simulink model "AFEsimpleModifsPV2"  (R2013a)
settings: Solver=FixedStepDiscrete  SolverMode=SingleTasking  StartTime=0.0  StopTime=5  FixedStep=Tpas  RelTol=1e-3
InitFcn:
  |  AFEsimpleparaDT1
values from neighbouring files (symbols this model uses):
  Freq = 50    [AFE_2L_RC_param_DT1.m]    (also in AFE_FV_Params.m; AFE_PontHPV2.m; AFEsimplepara.m; AFEsimpleparaDT1.m)
  hys = 100    [AFE_2L_RC_param_DT1.m]    (also in AFE_FV_Params.m = 150; AFE_PontHPV2.m = 150; AFEsimplepara.m = 0.1; AFEsimpleparaDT1.m)
  I = (P+Numd(2)/Dend(1))/Ts    [AFE_2L_RC_param_DT1.m]    (also in AFE_PontHPV2.m; AFEsimpleparaDT1.m; AFEsimpleparaPV2.m; initAFE_PontHPV3.m)
  Imax = 1300    [AFE_2L_RC_param_DT1.m]    (also in AFE_FV_Params.m = 1500; AFEsimpleparaDT1.m = 5000; AFEsimpleparaPV2.m = 5000)
  Lac = 8.1487e-04    (= 0.00081487)    [AFE_2L_RC_param_DT1.m]    (also in AFE_FV_Params.m; AFE_PontHPV2.m; AFEsimplepara.m = 0.002; AFEsimpleparaDT1.m)
  P = Numd(1)/Dend(1)    [AFE_2L_RC_param_DT1.m]    (also in AFE_PontHPV2.m; AFEsimpleparaDT1.m; AFEsimpleparaPV2.m; initAFE_PontHPV3.m)
  Rac = 2.5    [AFEsimplepara.m]
  Tpas = 5e-5    (= 5e-05)    [AFE_2L_RC_param_DT1.m]    (also in AFE_FV_Params.m; AFE_PontHPV2.m = 3e-06; AFEsimplepara.m = 1e-05; AFEsimpleparaDT1.m)
  Vac = 2000    [AFE_2L_RC_param_DT1.m]    (also in AFE_FV_Params.m; AFE_PontHPV2.m; AFEsimplepara.m; AFEsimpleparaDT1.m)
libraries: powerlib x16, powerlib_meascontrol x8, simulink x5
settings Model: Creator=LiberT  LastModifiedBy=Daniel
settings DataIOCC: SignalLoggingSaveFormat=ModelDataLogs
settings OptimizationCC: ExpressionDepthLimit=2147483647
settings DebuggingCC: MultiTaskDSMMsg=warning  MultiTaskCondExecSysMsg=none  FcnCallInpInsideContextMsg=EnableAllAsWarning  StrictBusMsg=None
settings RTWCC: IncludeERTFirstTime=on

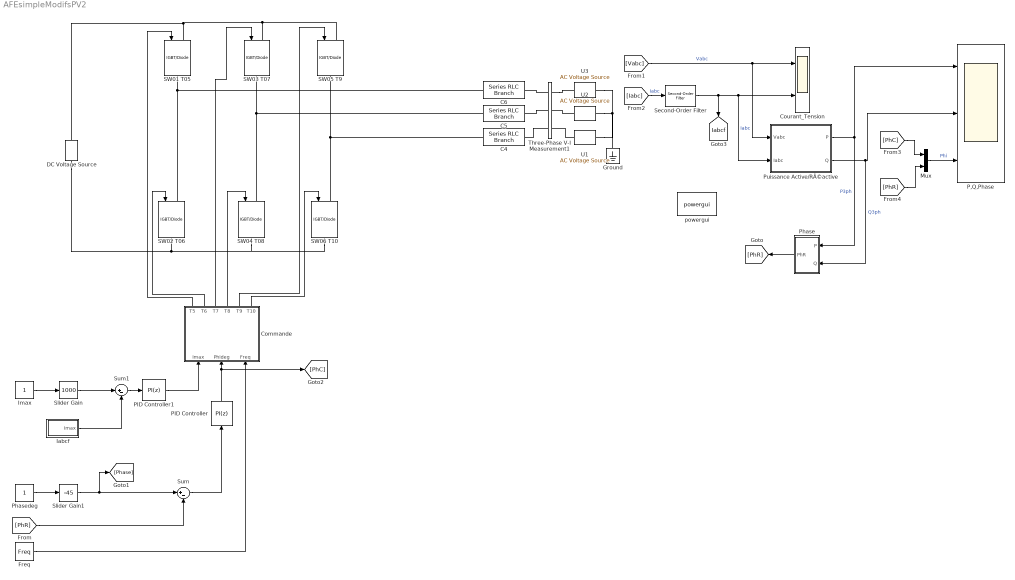
== system AFEsimpleModifsPV2 ==
  C4 : powerlib/Elements/Series RLC Branch  LConnTagsString=__new0  RConnTagsString=__new0  BranchType=L  Resistance=Rac  Inductance=Lac  SetiL0=off  InitialCurrent=0  Capacitance=300e-3  Setx0=off  InitialVoltage=0  Measurements=None
  C5 : powerlib/Elements/Series RLC Branch  LConnTagsString=__new0  RConnTagsString=__new0  BranchType=L  Resistance=Rac  Inductance=Lac  SetiL0=off  InitialCurrent=0  Capacitance=300e-3  Setx0=off  InitialVoltage=0  Measurements=None
  C6 : powerlib/Elements/Series RLC Branch  LConnTagsString=__new0  RConnTagsString=__new0  BranchType=L  Resistance=Rac  Inductance=Lac  SetiL0=off  InitialCurrent=0  Capacitance=300e-3  Setx0=off  InitialVoltage=0  Measurements=None
  Commande : Subsystem
  Courant_Tension : Scope  NumInputPorts=2
      settings: TickLabels=on  TimeRange=0.04  YMin=-1750~-2500  YMax=1750~2500  SaveName=Courant_Tension
  DC Voltage Source : powerlib/Electrical Sources/DC Voltage Source  Amplitude=5000  Measurements=None
  Freq : Constant  Value=Freq  SampleTime=Tpas
  Ground : powerlib/Elements/Ground  LConnTagsString=a
  Iabcf : Subsystem
  Imax : Constant  SampleTime=Tpas
  Mux : Mux  Inputs=2
  P,Q,Phase : Scope  NumInputPorts=3
      settings: TickLabels=on  TimeRange=5  YMin=-2.57e+06~-200000~-200  YMax=-2.45e+06~25000~200  SaveName=PQ_Phi  MaxDataPoints=50000
  PID Controller : simulink/Continuous/PID Controller  Controller=PI  TimeDomain=Discrete-time  SampleTime=Tpas  IntegratorMethod=Forward Euler  FilterMethod=Forward Euler  Form=Parallel  P=P  I=I  D=0  N=100  InitialConditionSource=internal  InitialConditionForIntegrator=0  InitialConditionForFilter=0  ExternalReset=none  LimitOutput=on  UpperSaturationLimit=179.5  LowerSaturationLimit=-179.5  LinearizeAsGain=on  AntiWindupMode=clamping  Kb=1  TrackingMode=off  Kt=1  PParamMin=[]  PParamMax=[]  IParamMin=[]  IParamMax=[]  DParamMin=[]  DParamMax=[]  NParamMin=[]  NParamMax=[]  KbParamMin=[]  KbParamMax=[]  KtParamMin=[]  KtParamMax=[]  POutMin=[]  POutMax=[]  IOutMin=[]  IOutMax=[]  DOutMin=[]  DOutMax=[]  NOutMin=[]  NOutMax=[]  KbOutMin=[]  KbOutMax=[]  KtOutMin=[]  KtOutMax=[]  IntegratorOutMin=[]  IntegratorOutMax=[]  FilterOutMin=[]  FilterOutMax=[]  SumOutMin=[]  SumOutMax=[]  SumI1OutMin=[]  SumI1OutMax=[]  SumI2OutMin=[]  SumI2OutMax=[]  SumI3OutMin=[]  SumI3OutMax=[]  SumDOutMin=[]  SumDOutMax=[]  SaturationOutMin=[]  SaturationOutMax=[]  IntegratorContinuousStateAttributes=''  IntegratorStateMustResolveToSignalObject=off  IntegratorRTWStateStorageClass=Auto  FilterContinuousStateAttributes=''  FilterStateMustResolveToSignalObject=off  FilterRTWStateStorageClass=Auto
  PID Controller1 : simulink/Continuous/PID Controller  Controller=PI  TimeDomain=Discrete-time  SampleTime=Tpas  IntegratorMethod=Forward Euler  FilterMethod=Forward Euler  Form=Parallel  P=5  I=20  D=0  N=100  InitialConditionSource=internal  InitialConditionForIntegrator=0  InitialConditionForFilter=0  ExternalReset=none  LimitOutput=on  UpperSaturationLimit=Imax  LowerSaturationLimit=0  LinearizeAsGain=on  AntiWindupMode=clamping  Kb=1  TrackingMode=off  Kt=1  PParamMin=[]  PParamMax=[]  IParamMin=[]  IParamMax=[]  DParamMin=[]  DParamMax=[]  NParamMin=[]  NParamMax=[]  KbParamMin=[]  KbParamMax=[]  KtParamMin=[]  KtParamMax=[]  POutMin=[]  POutMax=[]  IOutMin=[]  IOutMax=[]  DOutMin=[]  DOutMax=[]  NOutMin=[]  NOutMax=[]  KbOutMin=[]  KbOutMax=[]  KtOutMin=[]  KtOutMax=[]  IntegratorOutMin=[]  IntegratorOutMax=[]  FilterOutMin=[]  FilterOutMax=[]  SumOutMin=[]  SumOutMax=[]  SumI1OutMin=[]  SumI1OutMax=[]  SumI2OutMin=[]  SumI2OutMax=[]  SumI3OutMin=[]  SumI3OutMax=[]  SumDOutMin=[]  SumDOutMax=[]  SaturationOutMin=[]  SaturationOutMax=[]  IntegratorContinuousStateAttributes=''  IntegratorStateMustResolveToSignalObject=off  IntegratorRTWStateStorageClass=Auto  FilterContinuousStateAttributes=''  FilterStateMustResolveToSignalObject=off  FilterRTWStateStorageClass=Auto
  Phase : Subsystem
  Phasedeg : Constant  SampleTime=Tpas
  Puissance Active/RÃ©active : Subsystem
  SW01 T05 : powerlib/Power Electronics/IGBT//Diode  Ron=1e-3  Rs=1e5  Cs=Tpas  Measurements=off
  SW02 T06 : powerlib/Power Electronics/IGBT//Diode  Ron=1e-3  Rs=1e5  Cs=Tpas  Measurements=off
  SW03 T07 : powerlib/Power Electronics/IGBT//Diode  Ron=1e-3  Rs=1e5  Cs=Tpas  Measurements=off
  SW04 T08 : powerlib/Power Electronics/IGBT//Diode  Ron=1e-3  Rs=1e5  Cs=Tpas  Measurements=off
  SW05 T9 : powerlib/Power Electronics/IGBT//Diode  Ron=1e-3  Rs=1e5  Cs=Tpas  Measurements=off
  SW06 T10 : powerlib/Power Electronics/IGBT//Diode  Ron=1e-3  Rs=1e5  Cs=Tpas  Measurements=off
  Second-Order Filter : powerlib_meascontrol/Filters/Second-Order Filter  FilterType=Bandpass  Fo=50  Zeta=0.02  Ts=Tpas  Initialize=off  Vac_Init="[0,  0,  60]"  Vdc_Init=0  PlotResponse=off  FreqRange=[0, 500, 1]
  Slider Gain : simulink/Math Operations/Slider Gain  low=0  gain=1000  high=5000
  Slider Gain1 : simulink/Math Operations/Slider Gain  low=-180  gain=-45  high=180
  Sum : Sum  Inputs=|+-
  Sum1 : Sum  Inputs=|+-
  Three-Phase V-I Measurement1 : powerlib/Measurements/Three-Phase V-I Measurement  VoltageMeasurement=phase-to-ground  SetLabelV=on  LabelV=Vabc  Vpu=off  VpuLL=off  CurrentMeasurement=yes  SetLabelI=on  LabelI=Iabc  Ipu=off  Pbase=100e6  Vbase=500e3  OutputType=Complex  PhasorSimulation=off  PSBequivalent=0
  U1 : powerlib/Electrical Sources/AC Voltage Source  Amplitude=Vac*sqrt(2/3)  Phase=240  Frequency=Freq  SampleTime=0  Measurements=Voltage
  U2 : powerlib/Electrical Sources/AC Voltage Source  Amplitude=Vac*sqrt(2/3)  Phase=120  Frequency=Freq  SampleTime=0  Measurements=Voltage
  U3 : powerlib/Electrical Sources/AC Voltage Source  Amplitude=Vac*sqrt(2/3)  Phase=0  Frequency=Freq  SampleTime=0  Measurements=Voltage
  powergui : powerlib/powergui  Priority=1  SimulationMode=Discrete  SolverType=Tustin  SampleTime=Tpas  frequency=50  SPID=off  DisableSnubberDevices=off  DisableRonSwitches=off  DisableVfSwitches=off  SwTol=0  Interpol=off  DisplayEquations=off  frequencyindice=50  Pbase=100e6  ErrMax=1e-4  Iterations=50  UnitsV=kV  UnitsW=MW  FunctionMessages=off  echomessages=off  HookPort=off  EnableUseOfTLC=off  x0status=blocks  RestoreLinks=warning  ResistiveCurrentMeasurement=off  Frange=[0:2:500]  Ylog=off  Xlog=on  ShowGrid=off  save=off  variable=ZData  structure=ScopeData1  ZoomFFT=off  StartTime=8  cycles=100  DisplayStyle=1  fundamental=50  FreqAxis=off  MaxFrequency=100  frequencyindicesteady=1  RmsSteady=1  display=off  Ts=0  methode=off
  tag scope: Iabcf=global
  wires:
  [Iabc] -> Second-Order Filter/1  "Iabc"
  Commande/1(T5) -> SW01 T05/1
  Commande/2(T6) -> SW02 T06/1
  Commande/4(T8) -> SW04 T08/1
  Commande/3(T7) -> SW03 T07/1
  Commande/6(T10) -> SW06 T10/1
  Commande/5(T9) -> SW05 T9/1
  Freq/1 -> Commande/3(Freq)
  [Vabc] -> Courant_Tension/1, Puissance Active/RÃ©active/1(Vabc)  "Vabc"
  Puissance Active/RÃ©active/1(P) -> P,Q,Phase/1, Phase/1(P)  "P3ph"
  Imax/1 -> Slider Gain/1
  Phasedeg/1 -> Slider Gain1/1
  Second-Order Filter/1 -> [Iabcf], Courant_Tension/2, Puissance Active/RÃ©active/2(Iabc)  "Iabc"
  Slider Gain1/1 -> [Phase], Sum/1
  Phase/1(PhR) -> [PhR]
  [PhR] -> Sum/2
  [PhC] -> Mux/1
  [PhR] -> Mux/2
  Sum/1 -> PID Controller/1
  PID Controller/1 -> [PhC], Commande/2(Phideg)
  Mux/1 -> P,Q,Phase/3  "Phi"
  Puissance Active/RÃ©active/2(Q) -> Phase/2(Q), P,Q,Phase/2  "Q3ph"
  Slider Gain/1 -> Sum1/1
  Iabcf/1(Imax) -> Sum1/2
  Sum1/1 -> PID Controller1/1
  PID Controller1/1 -> Commande/1(Imax)
  connections:
  SW06 T10/RConn1 -- SW04 T08/RConn1 -- DC Voltage Source/LConn1 -- SW02 T06/RConn1
  SW01 T05/LConn1 -- DC Voltage Source/RConn1 -- SW05 T9/LConn1 -- SW03 T07/LConn1
  SW02 T06/LConn1 -- C6/LConn1 -- SW01 T05/RConn1
  SW06 T10/LConn1 -- SW05 T9/RConn1 -- C4/LConn1
  SW04 T08/LConn1 -- C5/LConn1 -- SW03 T07/RConn1
  U2/LConn1 -- U1/LConn1 -- Ground/LConn1 -- U3/LConn1
  Three-Phase V-I Measurement1/LConn1 -- C6/RConn1
  Three-Phase V-I Measurement1/RConn1 -- U3/RConn1
  U2/RConn1 -- Three-Phase V-I Measurement1/RConn2
  Three-Phase V-I Measurement1/LConn2 -- C5/RConn1
  C4/RConn1 -- Three-Phase V-I Measurement1/LConn3
  U1/RConn1 -- Three-Phase V-I Measurement1/RConn3

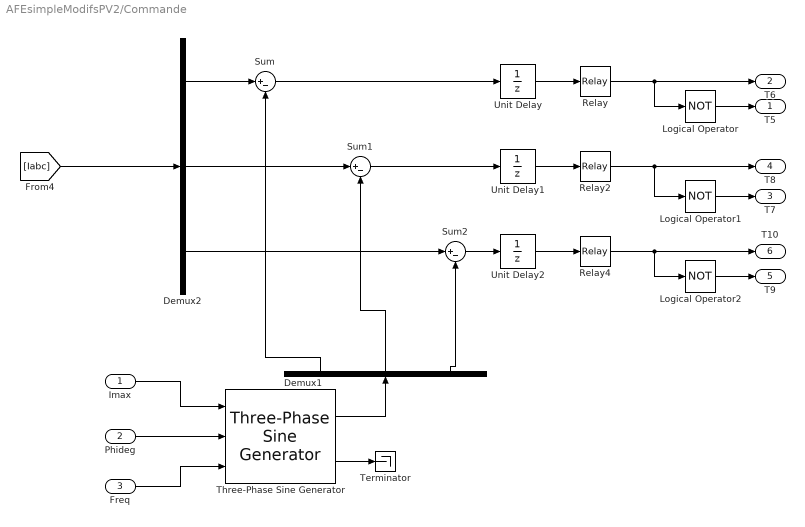
== system AFEsimpleModifsPV2/Commande ==
  Imax : Inport
  Phideg : Inport  Port=2
  Freq : Inport  Port=3
  Demux1 : Demux  Outputs=3
  Demux2 : Demux  Outputs=3
  Logical Operator : Logic  Operator=NOT  AllPortsSameDT=off
  Logical Operator1 : Logic  Operator=NOT  AllPortsSameDT=off
  Logical Operator2 : Logic  Operator=NOT  AllPortsSameDT=off
  Relay : Relay  OnSwitchValue=hys  OffSwitchValue=-hys
  Relay2 : Relay  OnSwitchValue=hys  OffSwitchValue=-hys
  Relay4 : Relay  OnSwitchValue=hys  OffSwitchValue=-hys
  Sum : Sum  Inputs=|+-
  Sum1 : Sum  Inputs=|+-
  Sum2 : Sum  Inputs=|+-
  Terminator : Terminator
  Three-Phase Sine Generator : powerlib_meascontrol/Pulse & Signal Generators/Three-Phase Sine Generator  Ts=Tpas
      link override Model/Discrete/Constant1: Value="[ 0  2*pi/3  -2*pi/3 ]"
  Unit Delay : UnitDelay  SampleTime=-1
  Unit Delay1 : UnitDelay  SampleTime=-1
  Unit Delay2 : UnitDelay  SampleTime=-1
  T5 : Outport
  T6 : Outport  Port=2
  T7 : Outport  Port=3
  T8 : Outport  Port=4
  T9 : Outport  Port=5
  T10 : Outport  Port=6
  wires:
  Demux2/1 -> Sum/1
  Demux2/2 -> Sum1/1
  Demux2/3 -> Sum2/1
  Sum/1 -> Unit Delay/1
  Sum1/1 -> Unit Delay1/1
  Sum2/1 -> Unit Delay2/1
  Unit Delay/1 -> Relay/1
  Unit Delay1/1 -> Relay2/1
  Unit Delay2/1 -> Relay4/1
  Logical Operator/1 -> T5/1
  Logical Operator1/1 -> T7/1
  Logical Operator2/1 -> T9/1
  Relay/1 -> T6/1, Logical Operator/1
  Relay2/1 -> T8/1, Logical Operator1/1
  Relay4/1 -> T10/1, Logical Operator2/1
  [Iabc] -> Demux2/1
  Imax/1 -> Three-Phase Sine Generator/1
  Freq/1 -> Three-Phase Sine Generator/3
  Three-Phase Sine Generator/1 -> Demux1/1
  Demux1/2 -> Sum1/2
  Demux1/3 -> Sum2/2
  Three-Phase Sine Generator/2 -> Terminator/1
  Phideg/1 -> Three-Phase Sine Generator/2
  Demux1/1 -> Sum/2

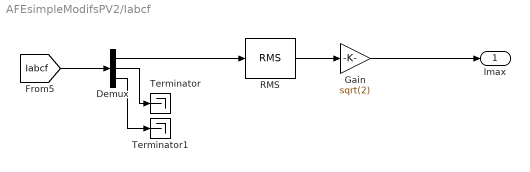
== system AFEsimpleModifsPV2/Iabcf ==
  Demux : Demux  Outputs=3
  Gain : Gain  Gain=sqrt(2)  SampleTime=Tpas
  RMS : powerlib_meascontrol/Measurements/RMS  TrueRMS=on  Freq=Freq  RMSInit=0  Ts=Tpas
  Terminator : Terminator
  Terminator1 : Terminator
  Imax : Outport
  wires:
  [Iabcf] -> Demux/1
  Demux/3 -> Terminator1/1
  Demux/2 -> Terminator/1
  Demux/1 -> RMS/1
  RMS/1 -> Gain/1
  Gain/1 -> Imax/1

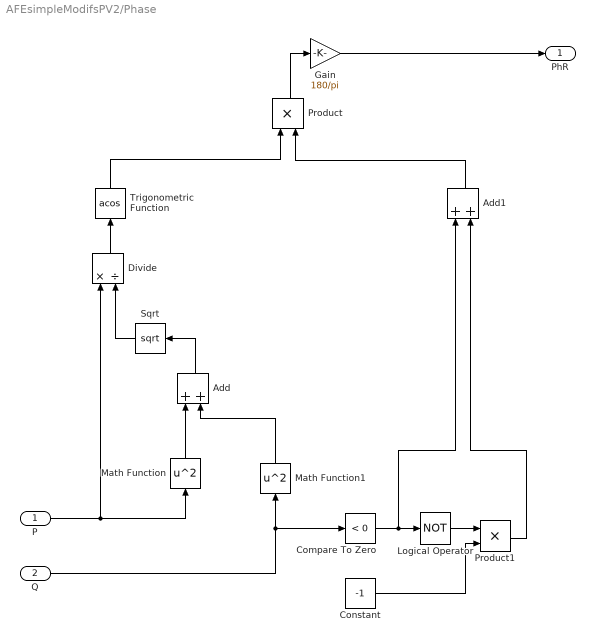
== system AFEsimpleModifsPV2/Phase ==
  P : Inport
  Q : Inport  Port=2
  Add : Sum
  Add1 : Sum  SampleTime=Tpas
  Compare To Zero : simulink/Logic and Bit Operations/Compare To Zero  relop=<  OutDataTypeStr=boolean
  Constant : Constant  Value=-1  SampleTime=Tpas
  Divide : Product  Inputs=*/
  Gain : Gain  Gain=180/pi  SampleTime=Tpas
  Logical Operator : Logic  Operator=NOT  AllPortsSameDT=off  OutDataTypeStr=boolean
  Math Function : Math  Operator=square  SampleTime=Tpas  SaturateOnIntegerOverflow=on
  Math Function1 : Math  Operator=square  SampleTime=Tpas  SaturateOnIntegerOverflow=on
  Product : Product
  Product1 : Product
  Sqrt : Sqrt  SaturateOnIntegerOverflow=on
  Trigonometric Function : Trigonometry  Operator=acos  SampleTime=Tpas
  PhR : Outport
  wires:
  P/1 -> Divide/1, Math Function/1
  Q/1 -> Math Function1/1, Compare To Zero/1
  Math Function/1 -> Add/1
  Math Function1/1 -> Add/2
  Add/1 -> Sqrt/1
  Sqrt/1 -> Divide/2
  Divide/1 -> Trigonometric Function/1
  Trigonometric Function/1 -> Product/1
  Compare To Zero/1 -> Add1/1, Logical Operator/1
  Logical Operator/1 -> Product1/1
  Constant/1 -> Product1/2
  Product1/1 -> Add1/2
  Add1/1 -> Product/2
  Product/1 -> Gain/1
  Gain/1 -> PhR/1

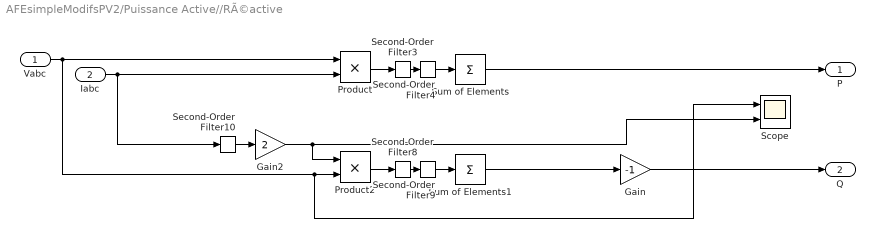
== system AFEsimpleModifsPV2/Puissance Active//RÃ©active ==
  Vabc : Inport
  Iabc : Inport  Port=2
  Gain : Gain  Gain=-1  SampleTime=Tpas
  Gain2 : Gain  Gain=2  SampleTime=Tpas
  Product : Product
  Product2 : Product
  Scope : Scope  NumInputPorts=2
      settings: YMin=-5~-5  YMax=5~5
  Second-Order Filter10 : powerlib_meascontrol/Filters/Second-Order Filter  FilterType=Lowpass  Fo=50  Zeta=1  Ts=Tpas  Initialize=off  Vac_Init="[0,  0,  60]"  Vdc_Init=0  PlotResponse=off  FreqRange=[0, 100, 1]
  Second-Order Filter3 : powerlib_meascontrol/Filters/Second-Order Filter  FilterType=Lowpass  Fo=10  Zeta=0.4  Ts=Tpas  Initialize=off  Vac_Init="[0,  0,  60]"  Vdc_Init=0  PlotResponse=off  FreqRange=[0, 200, 1]
  Second-Order Filter4 : powerlib_meascontrol/Filters/Second-Order Filter  FilterType=Lowpass  Fo=10  Zeta=1.1  Ts=Tpas  Initialize=off  Vac_Init="[0,  0,  60]"  Vdc_Init=0  PlotResponse=off  FreqRange=[0, 200, 1]
  Second-Order Filter8 : powerlib_meascontrol/Filters/Second-Order Filter  FilterType=Lowpass  Fo=10  Zeta=0.4  Ts=Tpas  Initialize=off  Vac_Init="[0,  0,  60]"  Vdc_Init=0  PlotResponse=off  FreqRange=[0, 200, 1]
  Second-Order Filter9 : powerlib_meascontrol/Filters/Second-Order Filter  FilterType=Lowpass  Fo=10  Zeta=1.1  Ts=Tpas  Initialize=off  Vac_Init="[0,  0,  60]"  Vdc_Init=0  PlotResponse=off  FreqRange=[0, 200, 1]
  Sum of Elements : Sum  Inputs=+
  Sum of Elements1 : Sum  Inputs=+
  P : Outport
  Q : Outport  Port=2
  wires:
  Second-Order Filter4/1 -> Sum of Elements/1
  Gain2/1 -> Scope/2, Product2/1
  Second-Order Filter3/1 -> Second-Order Filter4/1
  Product/1 -> Second-Order Filter3/1
  Sum of Elements/1 -> P/1
  Second-Order Filter8/1 -> Second-Order Filter9/1
  Product2/1 -> Second-Order Filter8/1
  Iabc/1 -> Second-Order Filter10/1, Product/2
  Vabc/1 -> Product/1, Scope/1, Product2/2
  Sum of Elements1/1 -> Gain/1
  Second-Order Filter10/1 -> Gain2/1
  Second-Order Filter9/1 -> Sum of Elements1/1
  Gain/1 -> Q/1
